simulink model "web_log"  (Simulink 7.3)
settings: Solver=ode3  SolverMode=SingleTasking  StartTime=0.0  StopTime=10.0  RelTol=1e-3
PreLoadFcn:
  | waijung.modelPreload; % Required for working with Waijung Blockset. Do not remove.
undefined symbols (not defined in the file): A0, A1, A2, A3, A7, B0, B1, B10, B11, B12, B13, Blocking, C1, C2, C3, C4, C5, HSEOSC, Link, LQFP176, Non, ST, STM32F417IG
libraries: simulink x45, amg_sqlite_dataserver x3, waijung_webserver x3, stm32f4_io_lib x1, stm32f4_device_config_lib x1
(part 1 of 3)
CloseFcn:
  | waijung.modelClose; % Required for working with Waijung Blockset. Do not remove.
settings Model: Creator=Krisada  LastModifiedBy=Krisada
settings OptimizationCC: OptimizeModelRefInitCode=on  LifeSpan=1
settings HardwareCC: ProdEndianess=LittleEndian  ProdHWDeviceType=ARM Compatible->Cortex - M4  TargetEndianess=LittleEndian  TargetHWDeviceType=ARM Compatible->Cortex - M4
settings RTWCC: SystemTargetFile=stm32f4.tlc  GenerateMakefile=off  TemplateMakefile=ert_default_tmf  Description=STM32F4 Target  ProcessScript=stm32f4_make_rtw_hook
settings CodeAppCC: IgnoreCustomStorageClasses=off
settings STFCustomTargetCC: ModelReferenceCompliant=off  CombineOutputUpdateFcns=on  ERTCustomFileBanners=on  SupportContinuousTime=off  SupportNonInlinedSFcns=off  SystemTargetFile=stm32f4.tlc
settings ERTTargetCC: MultiwordLength=2048  ModelReferenceCompliant=off  ParMdlRefBuildCompliant=off  CompOptLevelCompliant=off  ERTFirstTimeCompliant=off  ModelStepFunctionPrototypeControlCompliant=off  CPPClassGenCompliant=off  InlinedParameterPlacement=NonHierarchical  ERTSrcFileBannerTemplate=stm32f4_code_template.cgt  ERTHdrFileBannerTemplate=stm32f4_code_template.cgt  ERTDataSrcFileTemplate=stm32f4_code_template.cgt  ERTDataHdrFileTemplate=stm32f4_code_template.cgt  ERTCustomFileTemplate=stm32f4_file_process.tlc

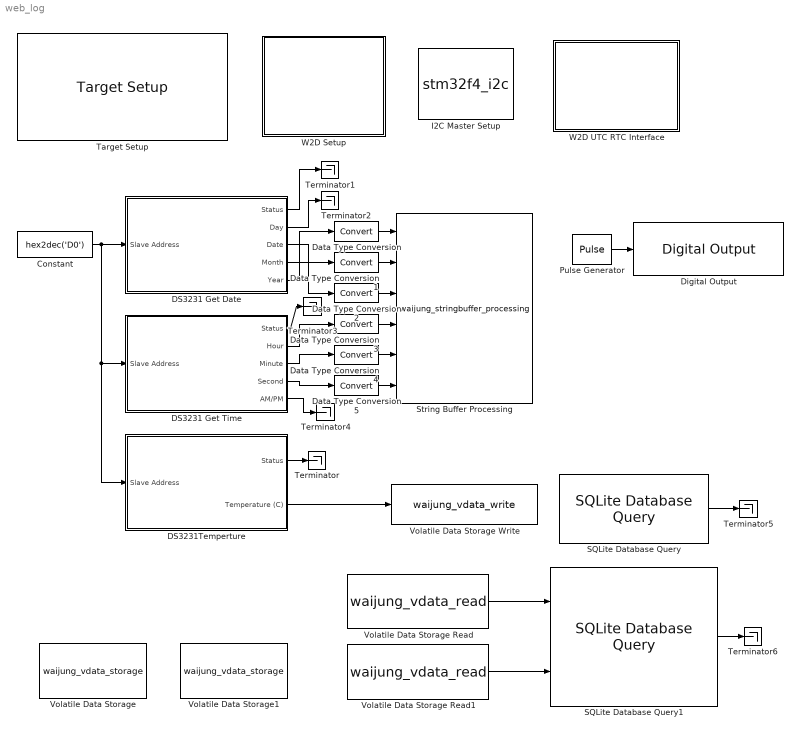
== system web_log ==
  Constant : Constant  Value=hex2dec('D0')  OutDataTypeMode=uint8  OutDataType=fixdt(1, 16)  OutScaling=2^0  OutDataTypeStr=uint8
  DS3231 Get Date : Subsystem  mask{blockfunction=date, module=1}
      mask prompts: blockfunction "Function"; module "I2C module"
      mask init:
      | amg_high_precision_rtc_callback('init');
      mask Help: web(fullfile(waijungdocroot,'DS3231_Get_Date.htm'), '-browser')
      mask StyleString: popup(temp|time|date),popup(1|2|3)
      mask CallbackString: |amg_high_precision_rtc_callback('module');
      mask Display: text(0.5, 0.5, 'Port: I2C1','ver','middle','hor','center');port_label('input', 1,'SlvAddr');port_label('output', 1,'Status');port_label('output', 2,'Day(1-7)');port_label('output', 3,'Date(1-31)');port_label('output', 4,'Month(1-12)');port_label('output', 5,'Year(0-99)');
  DS3231 Get Time : Subsystem  mask{blockfunction=time, module=1}
      mask prompts: blockfunction "Function"; module "I2C module"
      mask init:
      | amg_high_precision_rtc_callback('init');
      mask Help: web(fullfile(waijungdocroot,'DS3231_Get_Time.htm'), '-browser')
      mask StyleString: popup(temp|time|date),popup(1|2|3)
      mask CallbackString: |amg_high_precision_rtc_callback('module');
      mask Display: text(0.5, 0.5, 'Port: I2C1','ver','middle','hor','center');port_label('input', 1,'SlvAddr');port_label('output', 1,'Status');port_label('output', 2,'Hour(0-11/23)');port_label('output', 3,'Minute(0-59)');port_label('output', 4,'Second(0-59)');port_label('output', 5,'AM(0)/PM(1)');
  DS3231Temperture : Subsystem  mask{blockfunction=temp, module=1}
      mask prompts: blockfunction "Function"; module "I2C module"
      mask help:
      | The block implement temperature reading from DS3231 (Extremely Accurate RTC).
      | Its override the CONV bit, to force the temperature update, so the recommend sample time for this block is more than 0.5 seconds.
      | To get reading value from DS3231 device, this block generate 3 transaction of I2C as below:
      | 1. Read 2 bytes data from register 0x11 and 0x12 (Sequential read).
      | 2. Read 1 byte data from register 0x0F (Status) for poll BSY bit.
      | 3. Write 1 byte data to register 0x0E to force temperature conversion, CONV bit.
      mask init:
      | amg_high_precision_rtc_callback('init');
      mask Help: web(fullfile(waijungdocroot,'DS3231Temperture.htm'), '-browser')
      mask StyleString: popup(temp|time|date),popup(1|2|3)
      mask CallbackString: |amg_high_precision_rtc_callback('module');
      mask Display: text(0.5, 0.5, 'Port: I2C1','ver','middle','hor','center');port_label('input', 1,'SlvAddr');port_label('output', 1,'Status');port_label('output', 2,'Temp (C)');
  Data Type Conversion{,1..5} (6 alike) : DataTypeConversion  OutDataType=fixdt(1, 16)  OutScaling=2^0
  Digital Output : stm32f4_io_lib/Digital Output  use_bitband=on  port=D  speed=100  porttype=Push Pull  porttypestr=PP  use_pin0=off  use_pin1=off  use_pin2=off  use_pin3=off  use_pin4=off  use_pin5=off  use_pin6=off  use_pin7=off  use_pin8=off  use_pin9=off  use_pin10=off  use_pin11=off  use_pin12=on  use_pin13=off  use_pin14=off  use_pin15=off  pinstr=GPIO_Pin_12  usedpinarray="[0  0  0  0  0  0  0  0  0  0  0  0  1  0  0  0]"  bitbandingstr="#define DigitalOutput_D12 Peripheral_BB(GPIOD->ODR, 12)  /* Output pin */"  sampletime=-1  sampletimestr=0.25  blockid=DigitalOutput  enablecustomportlabel=off  globalinit=off  cinputportlabel=In1, In2  coutputportlabel=0
  I2C Master Setup : S-Function  FunctionName=stm32f4_i2c  Parameters=configuration,module,transfer,clkspeed,timeout,sdapin,sclpin,writecount,readcount,inputtypearray,outputtypearray,confstr,sampletime,sampletimestr,blockid  EnableBusSupport=off  mask(stm32f4_i2c){configuration=Setup, module=1, lastmodule=1, transfer=Blocking, dutycycle=TLow/THigh = 2, clkspeed=400, timeout=25, writecount=0, readcount=0, sdapin=B7, sclpin=B6, waitwritetime=0, inputtypearray=[0], outputtypearray=[0], confstr=["B","7","B","6","1","1","6","0","I2C_DutyCycle_2","0","off"], sampletime=-1, sampletimestr=0.001, blockid=I2CMasterSetup}
      mask prompts: module "I2C Module"; lastmodule "Last module"; transfer "Transfer mode"; dutycycle "Duty cycle in fast mode"; clkspeed "Clock speed (kHz)"; timeout "Timeout (ms)"; writecount "Bytes write count"; readcount "Bytes read count"; sdapin "SDA pin"; sclpin "SCL pin"; waitwritetime "Wait write time (ms), default is 0"; inputtypearray "Input type array"; outputtypearray "Output type array"; confstr "Configuration string"; sampletime "Sample time (sec)"; sampletimestr "Compiled sample time (sec) in string"
      mask init:
      | stm32f4_i2c_callback('init');
      mask Help: web(fullfile(waijungdocroot,'stm32f4_i2c_setup.htm'), '-browser')
      mask StyleString: popup(Setup|Transaction),popup(1|2|3),edit,popup(Blocking|Non-blocking),popup(TLow/THigh = 16/9|TLow/THigh = 2),edit,edit,edit,edit,popup(Not used|B7|B9),popup(Not used|B6|B8),edit,edit,edit,edit,edit,edit,edit
      mask CallbackString: stm32f4_i2c_callback('configuration');|stm32f4_i2c_callback('module');|||stm32f4_i2c_callback('dutycycle');|||stm32f4_i2c_callback('writecount');|stm32f4_i2c_callback('readcount');|stm32f4_i2c_callback('sdapin');|stm32f4_i2c_callback('sclpin');||||stm32f4_i2c_callback('confstr');|stm32f4_i2c_callback('sampletime');|stm32f4_i2c_callback('sampletimestr');|stm32f4_i2c_callback('blockid');
      mask Display: text(0.5, 0.5, 'Module: I2C1\nClock: 400kHz\nSDA/SCL Pin: B7/B6','ver','middle','hor','center');
  Pulse Generator : DiscretePulseGenerator  PulseType=Time based  Amplitude=1  Period=0.5  PulseWidth=50  PhaseDelay=0  SampleTime=1
  SQLite Database Query : amg_sqlite_dataserver/SQLite Database Query  Priority=1  transfer=Non-Blocking  statement=CREATE  filenameoption=Specific  filename='database.db'  tablenameoption=Specific  tablename='logging'  columns='time text,temp real'  condition='where rowid==1'  preview=CREATE TABLE IF NOT EXISTS %s(time text,temp real);  enablestatus=on  columncount=2  columnnamesarray="[\"time\",\"temp\"]"  columntypesarray="[\"string\",\"single\"]"  inputtypearray=[]  outputtypearray=[7]  sampletime=inf  sampletimestr=0.001  blockid=SQLiteDatabaseQuery
  SQLite Database Query1 : amg_sqlite_dataserver/SQLite Database Query  Priority=5  transfer=Non-Blocking  statement=INSERT  filenameoption=Specific  filename='database.db'  tablenameoption=Specific  tablename='logging'  columns='time text,temp real'  condition='where rowid==1'  preview=INSERT INTO %s (time,temp)VALUES('%s',%f);  enablestatus=on  columncount=2  columnnamesarray="[\"time\",\"temp\"]"  columntypesarray="[\"string\",\"single\"]"  inputtypearray=[7 1]  outputtypearray=[7]  sampletime=30  sampletimestr=30  blockid=SQLiteDatabaseQuery1
  String Buffer Processing : S-Function  Priority=1  FunctionName=waijung_stringbuffer_processing  Parameters=configuration,varname,sformat,porttypes,portcount,inputtypearray,outputtypearray,sampletime,sampletimestr,blockid  EnableBusSupport=off  mask(waijung_stringbuffer_processing){configuration=sprintf, storagename=timestring, sformat='%02d%02d%02d%02d%02d%02d', enableoutput=off, varname=VolatileDataStorage_timestring, inputtypearray=[6 -1 -1 -1 -1 -1 -1], outputtypearray=[0], porttypes=["int32_t","int32_t","int32_t","int32_t","int32_t","int32_t"], portcount=6, sampletime=1, sampletimestr=1, blockid=StringBufferProcessing}
      mask prompts: configuration "Function"; storagename "String buffer"; sformat "Printf format"; enableoutput "Enable output status"; varname "Variable name"; inputtypearray "Input type array"; outputtypearray "Output type array"; porttypes "Port type list"; portcount "Port type count"; sampletime "Sample time (sec)"; sampletimestr "Compiled sample time (sec) in string"
      mask help:
      | This block implements string processing, sprintf/ sscanf command.
      | Supported format:
      | %u, %i, %o, %x: uint32
      | %d: int32
      | %e, %g, %f: single
      | %c: int8
      |
      | Status:
      |  0: Failed.
      |  Non-zero: Success.
      mask init:
      | waijung_stringbuffer_processing_callback('init');
      mask Help: web(fullfile(waijungdocroot,'String_Buffer_Processing.htm'))
      mask StyleString: popup(sprintf|sscanf),popup(timestring|date|time|mcutime|browsertime|<output>),edit,checkbox,edit,edit,edit,edit,edit,edit,edit,edit
      mask CallbackString: waijung_stringbuffer_processing_callback('configuration');||waijung_stringbuffer_processing_callback('sformat');|waijung_stringbuffer_processing_callback('enableoutput');||||||waijung_stringbuffer_processing_callback('sampletime');|waijung_stringbuffer_processing_callback('sampletimestr');|waijung_stringbuffer_processing_callback('blockid');
      mask Display: text(0.5, 0.5, '[ sprintf ]\nBuffer: timestring\nTs (sec): 1','ver','middle','hor','center');port_label('input', 1,'%d');port_label('input', 2,'%d');port_label('input', 3,'%d');port_label('input', 4,'%d');port_label('input', 5,'%d');port_label('input', 6,'%d');
  Target Setup : stm32f4_device_config_lib/Target Setup  Priority=100  compiler=GNU ARM  previous_compiler=GNU ARM  mcu=STM32F417IG (LQFP176)  mcustr=STM32F417IG  clockconfig=HSEOSC-8MHz  system_stm32f4xx_c_path=F:\trunk\targets\stm32f4_target\stm32f4\utils\system_stm32f4xx_default\STM32F40_41xxx\hseosc8mhz  showmemoryconfiguration=on  stacksize=0x2000  heapsize=0x4000  enableautocompiledownload=on  fullchiperase=off  programmerinterface=ST-Link  editctrlstr=on  compilercontrolstr=$(patsubst %, -I%, .) -mcpu=cortex-m4 -mthumb -mthumb-interwork -mfloat-abi=hard -mfpu=fpv4-sp-d16 -ffast-math -Wall -Wextra -Ofast  assemblercontrolstr=$(patsubst %, -I%, .) -mcpu=cortex-m4 -mthumb -mthumb-interwork -mfloat-abi=hard -mfpu=fpv4-sp-d16 -ffast-math -Wall -Wextra -Ofast -Wa,-amhls=$(<:.s=.lst) -D__STACK_SIZE=$(STACK_SIZE) -D__HEAP_SIZE=$(HEAP_SIZE)  linkercontrolstr=-T$(LD_SCRIPT) -g -Wl,-Map=$(MAP),--cref,--no-warn-mismatch -mcpu=cortex-m4 -mthumb -mthumb-interwork -mfloat-abi=hard -mfpu=fpv4-sp-d16 -specs=nosys.specs  runafterdownload=on  execprofile=None  profileruart=3  profilerbaud=500000  profilertxpin=D8  profilerinitstr=0.001,168000000,168000,500000,0  manualsetsampletime=off  sampletime=0.001  blockid=TargetSetup  systickreloadvalue=168000  hseval=8000000  lastprofileruart=3  hclk=168000000  flashorigin=0x8000000  flashlength=1024k  ramorigin=0x20000000  ramlength=128k  useextram=off
  Terminator{,1..6} (7 alike) : Terminator
  Volatile Data Storage : S-Function  FunctionName=waijung_vdata_storage  Parameters=storagetype,storagename,initval,varname,buffersize,initvalstring,sampletime,sampletimestr,blockid,storagetypestr  EnableBusSupport=off  mask(waijung_vdata_storage){storagetype=string, storagename=timestring, initval=0, varname=VolatileDataStorage_timestring, buffersize=64, initvalstring='Initial string', webintegration=ReadOnly with KeyValuePair, weboutputformat='%s', webcgicallback=(void*)0, laststoragetype=string, sampletime=-1, sampletimestr=0.001, blockid=VolatileDataStorage, storagetypestr=char}
      mask prompts: storagetype "Storage Type"; storagename "Storage Name (must be a valid variable name)"; initval "Initial value (Apply at Power on Reset only)"; varname "Variable name"; buffersize "Size (bytes)"; initvalstring "Initial value (Apply at Power on Reset only)"; webintegration "Web CGI varget/varset integration"; weboutputformat "Web CGI varget output format"; webcgicallback "Web CGI varset callback"; laststoragetype "Last selected Storage Type"; sampletime "Sample time (sec)"; sampletimestr "Compiled sample time (sec) in string"; storagetypestr "Type string"
      mask help:
      | This block implements a volatile Data Storage.
      |
      | Web CGI varset/varget integratiopn:
      | Enable - In webserver application, allow remote access via http.
      | Disable - Variable is use in local only.
      mask init:
      | waijung_vdata_storage_callback('init');
      mask Help: web(fullfile(waijungdocroot,'Volatile_Data_Storage.htm'))
      mask StyleString: popup(double|single|uint32|int32|uint16|int16|uint8|int8|string),edit,edit,edit,edit,edit,popup(Disable|ReadOnly|Write/ Read|ReadOnly with KeyValuePair|Write/ Read with KeyValuePair),edit,edit,popup(double|single|uint32|int32|uint16|int16|uint8|int8|string),edit,edit,edit,edit
      mask CallbackString: waijung_vdata_storage_callback('storagetype');|waijung_vdata_storage_callback('storagename');|waijung_vdata_storage_callback('initval');|waijung_vdata_storage_callback('varname');||waijung_vdata_storage_callback('initvalstring');|waijung_vdata_storage_callback('webintegration');|waijung_vdata_storage_callback('weboutputformat');|||waijung_vdata_storage_callback('sampletime');|waijung_vdata_storage_callback('sampletimestr');|waijung_vdata_storage_callback('blockid');|
      mask Display: text(0.5, 0.5, 'Name: timestring\nType: string','ver','middle','hor','center')
  Volatile Data Storage Read : S-Function  FunctionName=waijung_vdata_read  Parameters=storagename,varname,sampletime,sampletimestr,blockid,storagetype,storagetypestr  EnableBusSupport=off  mask(waijung_vdata_read){storagename=timestring, varname=VolatileDataStorage_timestring, sampletime=inf, sampletimestr=30, blockid=VolatileDataStorageRead, storagetype=string, storagetypestr=uint32_t}
      mask prompts: storagename "Storage Name"; varname "Variable name"; sampletime "Sample time (sec)"; sampletimestr "Compiled sample time (sec) in string"; storagetype "Data type"; storagetypestr "Data type string"
      mask help: This block implements read data from a buffer.
      mask init:
      | waijung_vdata_read_callback('init');
      mask Help: web(fullfile(waijungdocroot,'Volatile_Data_Storage_Read.htm'))
      mask StyleString: popup(timestring|temperature|date|time|mcutime|browsertime|minth|hourth|secth),edit,edit,edit,edit,edit,edit
      mask CallbackString: waijung_vdata_read_callback('storagename');|waijung_vdata_read_callback('varname');|waijung_vdata_read_callback('sampletime');|waijung_vdata_read_callback('sampletimestr');|waijung_vdata_read_callback('blockid');|waijung_vdata_read_callback('storagetype');|
      mask Display: text(0.05, 0.5, 'Buffer: timestring','ver','middle','hor','left');port_label('output',1,'D1(string)')
  Volatile Data Storage Read1 : S-Function  FunctionName=waijung_vdata_read  Parameters=storagename,varname,sampletime,sampletimestr,blockid,storagetype,storagetypestr  EnableBusSupport=off  mask(waijung_vdata_read){storagename=temperature, varname=VolatileDataStorage1_temperature, sampletime=inf, sampletimestr=30, blockid=VolatileDataStorageRead1, storagetype=single, storagetypestr=float}
      mask prompts: storagename "Storage Name"; varname "Variable name"; sampletime "Sample time (sec)"; sampletimestr "Compiled sample time (sec) in string"; storagetype "Data type"; storagetypestr "Data type string"
      mask help: This block implements read data from a buffer.
      mask init:
      | waijung_vdata_read_callback('init');
      mask Help: web(fullfile(waijungdocroot,'Volatile_Data_Storage_Read.htm'))
      mask StyleString: popup(timestring|temperature|date|time|mcutime|browsertime|minth|hourth|secth),edit,edit,edit,edit,edit,edit
      mask CallbackString: waijung_vdata_read_callback('storagename');|waijung_vdata_read_callback('varname');|waijung_vdata_read_callback('sampletime');|waijung_vdata_read_callback('sampletimestr');|waijung_vdata_read_callback('blockid');|waijung_vdata_read_callback('storagetype');|
      mask Display: text(0.05, 0.5, 'Buffer: temperature','ver','middle','hor','left');port_label('output',1,'D1(single)')
  Volatile Data Storage Write : S-Function  FunctionName=waijung_vdata_write  Parameters=storagename,varname,sampletime,sampletimestr,blockid,storagetype,storagetypestr  EnableBusSupport=off  mask(waijung_vdata_write){storagename=temperature, varname=VolatileDataStorage1_temperature, sampletime=-1, sampletimestr=1, blockid=VolatileDataStorageWrite, storagetype=single, storagetypestr=float}
      mask prompts: storagename "Storage Name"; varname "Variable name"; sampletime "Sample time (sec)"; sampletimestr "Compiled sample time (sec) in string"; storagetype "Data type"; storagetypestr "Data type string"
      mask help: This block implements write data to a buffer.
      mask init:
      | waijung_vdata_write_callback('init');
      mask Help: web(fullfile(waijungdocroot,'Volatile_Data_Storage_Write.htm'))
      mask StyleString: popup(timestring|temperature|date|time|mcutime|browsertime|minth|hourth|secth),edit,edit,edit,edit,edit,edit
      mask CallbackString: waijung_vdata_write_callback('storagename');|waijung_vdata_write_callback('varname');|waijung_vdata_write_callback('sampletime');|waijung_vdata_write_callback('sampletimestr');|waijung_vdata_write_callback('blockid');|waijung_vdata_write_callback('storagetype');|
      mask Display: text(0.95, 0.5, 'Buffer: temperature','ver','middle','hor','right');port_label('input',1,'D1(single)')
  Volatile Data Storage1 : S-Function  FunctionName=waijung_vdata_storage  Parameters=storagetype,storagename,initval,varname,buffersize,initvalstring,sampletime,sampletimestr,blockid,storagetypestr  EnableBusSupport=off  mask(waijung_vdata_storage){storagetype=single, storagename=temperature, initval=0, varname=VolatileDataStorage1_temperature, buffersize=64, initvalstring='Initial string', webintegration=ReadOnly with KeyValuePair, weboutputformat='%f', webcgicallback=(void*)0, laststoragetype=single, sampletime=-1, sampletimestr=0.001, blockid=VolatileDataStorage1, storagetypestr=float}
      mask prompts: storagetype "Storage Type"; storagename "Storage Name (must be a valid variable name)"; initval "Initial value (Apply at Power on Reset only)"; varname "Variable name"; buffersize "Size (bytes)"; initvalstring "Initial value (Apply at Power on Reset only)"; webintegration "Web CGI varget/varset integration"; weboutputformat "Web CGI varget output format"; webcgicallback "Web CGI varset callback"; laststoragetype "Last selected Storage Type"; sampletime "Sample time (sec)"; sampletimestr "Compiled sample time (sec) in string"; storagetypestr "Type string"
      mask help:
      | This block implements a volatile Data Storage.
      |
      | Web CGI varset/varget integratiopn:
      | Enable - In webserver application, allow remote access via http.
      | Disable - Variable is use in local only.
      mask init:
      | waijung_vdata_storage_callback('init');
      mask Help: web(fullfile(waijungdocroot,'Volatile_Data_Storage.htm'))
      mask StyleString: popup(double|single|uint32|int32|uint16|int16|uint8|int8|string),edit,edit,edit,edit,edit,popup(Disable|ReadOnly|Write/ Read|ReadOnly with KeyValuePair|Write/ Read with KeyValuePair),edit,edit,popup(double|single|uint32|int32|uint16|int16|uint8|int8|string),edit,edit,edit,edit
      mask CallbackString: waijung_vdata_storage_callback('storagetype');|waijung_vdata_storage_callback('storagename');|waijung_vdata_storage_callback('initval');|waijung_vdata_storage_callback('varname');||waijung_vdata_storage_callback('initvalstring');|waijung_vdata_storage_callback('webintegration');|waijung_vdata_storage_callback('weboutputformat');|||waijung_vdata_storage_callback('sampletime');|waijung_vdata_storage_callback('sampletimestr');|waijung_vdata_storage_callback('blockid');|
      mask Display: text(0.5, 0.5, 'Name: temperature\nType: single','ver','middle','hor','center')
  W2D Setup : Subsystem
  W2D UTC RTC Interface : Subsystem  Priority=1
  wires:
  Pulse Generator/1 -> Digital Output/1
  Constant/1 -> DS3231 Get Date/1(Slave Address), DS3231 Get Time/1(Slave Address), DS3231Temperture/1(Slave Address)
  DS3231Temperture/1(Status) -> Terminator/1
  DS3231Temperture/2(Temperature (C)) -> Volatile Data Storage Write/1
  Data Type Conversion/1 -> String Buffer Processing/1
  Data Type Conversion1/1 -> String Buffer Processing/2
  Data Type Conversion2/1 -> String Buffer Processing/3
  Data Type Conversion3/1 -> String Buffer Processing/4
  Data Type Conversion4/1 -> String Buffer Processing/5
  Data Type Conversion5/1 -> String Buffer Processing/6
  DS3231 Get Date/5(Year) -> Data Type Conversion/1
  DS3231 Get Date/4(Month) -> Data Type Conversion1/1
  DS3231 Get Date/3(Date) -> Data Type Conversion2/1
  DS3231 Get Time/2(Hour) -> Data Type Conversion3/1
  DS3231 Get Time/3(Minute) -> Data Type Conversion4/1
  DS3231 Get Time/4(Second) -> Data Type Conversion5/1
  DS3231 Get Date/1(Status) -> Terminator1/1
  DS3231 Get Date/2(Day) -> Terminator2/1
  DS3231 Get Time/1(Status) -> Terminator3/1
  DS3231 Get Time/5(AM/PM) -> Terminator4/1
  SQLite Database Query/1 -> Terminator5/1
  SQLite Database Query1/1 -> Terminator6/1
  Volatile Data Storage Read/1 -> SQLite Database Query1/1
  Volatile Data Storage Read1/1 -> SQLite Database Query1/2

== system web_log/DS3231 Get Date ==
  Slave Address : Inport  OutDataType=fixdt(1, 16)  OutScaling=2^0
  Compare To Zero : simulink/Logic and Bit Operations/Compare To Zero  SystemSampleTime=-1  relop===  LogicOutDataTypeMode=uint8  ZeroCross=off
  Convert : Subsystem  TreatAsAtomicUnit=on
  I2C Master Read/Write : S-Function  FunctionName=stm32f4_i2c  Parameters=configuration,module,transfer,clkspeed,timeout,sdapin,sclpin,writecount,readcount,inputtypearray,outputtypearray,confstr,sampletime,sampletimestr,blockid  EnableBusSupport=off  mask(stm32f4_i2c){configuration=Transaction, module=1, lastmodule=3, transfer=Blocking, dutycycle=TLow/THigh = 2, clkspeed=400, timeout=25, writecount=1, readcount=4, sdapin=C9, sclpin=A8, waitwritetime=0, inputtypearray=[2 3 3], outputtypearray=[5 3 3 3 3 3], confstr=["C","9","A","8","1","1","6","0","I2C_DutyCycle_2","0","off"], sampletime=-1, sampletimestr=1, blockid=DS3231GetDateI2CMasterReadWrite}
      mask prompts: module "I2C Module"; lastmodule "Last module"; transfer "Transfer mode"; dutycycle "Duty cycle in fast mode"; clkspeed "Clock speed (kHz)"; timeout "Timeout (ms)"; writecount "Bytes write count"; readcount "Bytes read count"; sdapin "SDA pin"; sclpin "SCL pin"; waitwritetime "Wait write time (ms), default is 0"; inputtypearray "Input type array"; outputtypearray "Output type array"; confstr "Configuration string"; sampletime "Sample time (sec)"; sampletimestr "Compiled sample time (sec) in string"
      mask init:
      | stm32f4_i2c_callback('init');
      mask Help: web(fullfile(waijungdocroot,'stm32f4_i2c_readwrite.htm'), '-browser')
      mask StyleString: popup(Setup|Transaction),popup(1|2|3),edit,popup(Blocking|Non-blocking),popup(TLow/THigh = 16/9|TLow/THigh = 2),edit,edit,edit,edit,popup(-|C9),popup(-|A8),edit,edit,edit,edit,edit,edit,edit
      mask CallbackString: stm32f4_i2c_callback('configuration');|stm32f4_i2c_callback('module');|||stm32f4_i2c_callback('dutycycle');|||stm32f4_i2c_callback('writecount');|stm32f4_i2c_callback('readcount');|stm32f4_i2c_callback('sdapin');|stm32f4_i2c_callback('sclpin');||||stm32f4_i2c_callback('confstr');|stm32f4_i2c_callback('sampletime');|stm32f4_i2c_callback('sampletimestr');|stm32f4_i2c_callback('blockid');
      mask Display: text(0.5, 0.5, 'Module: I2C1\nTransfer: Blocking\nWrite: 1 bytes\nRead: 4 bytes\nTs (sec): 1','ver','middle','hor','center');port_label('input', 1,'SlvAddr');port_label('input', 2,'Wr0 (uint8)');port_label('output', 1,'Status');port_label('output', 2,'Rd0 (uint8)');port_label('output', 3,'Rd1 (uint8)');port_label('output', 4,'Rd2 (uint8)');port_label('output', 5,'Rd3 (uint8)');
  REG_DATE : Constant  Value=hex2dec('03')  OutDataTypeMode=uint8  OutDataType=fixdt(1, 16)  OutScaling=2^0  OutDataTypeStr=uint8
  Status : Outport
  Day : Outport  Port=2
  Date : Outport  Port=3
  Month : Outport  Port=4
  Year : Outport  Port=5
  wires:
  Convert/3(Month) -> Month/1
  Convert/4(Year) -> Year/1
  Convert/2(Date) -> Date/1
  Convert/1(Day) -> Day/1
  I2C Master Read/Write/5 -> Convert/4(In4)
  REG_DATE/1 -> I2C Master Read/Write/2
  Slave Address/1 -> I2C Master Read/Write/1
  I2C Master Read/Write/1 -> Compare To Zero/1
  Compare To Zero/1 -> Convert/Enable, Status/1
  I2C Master Read/Write/2 -> Convert/1(In1)
  I2C Master Read/Write/3 -> Convert/2(In2)
  I2C Master Read/Write/4 -> Convert/3(In3)

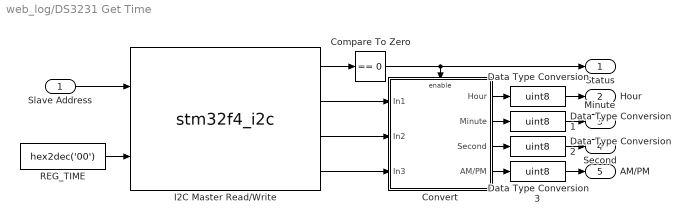
== system web_log/DS3231 Get Time ==
  Slave Address : Inport  OutDataType=fixdt(1, 16)  OutScaling=2^0
  Compare To Zero : simulink/Logic and Bit Operations/Compare To Zero  SystemSampleTime=-1  relop===  LogicOutDataTypeMode=uint8  ZeroCross=off
  Convert : Subsystem  TreatAsAtomicUnit=on
  Data Type Conversion{,1..3} (4 alike) : DataTypeConversion  OutDataTypeMode=uint8  OutDataType=fixdt(1, 16)  OutScaling=2^0  OutDataTypeStr=uint8
  I2C Master Read/Write : S-Function  FunctionName=stm32f4_i2c  Parameters=configuration,module,transfer,clkspeed,timeout,sdapin,sclpin,writecount,readcount,inputtypearray,outputtypearray,confstr,sampletime,sampletimestr,blockid  EnableBusSupport=off  mask(stm32f4_i2c){configuration=Transaction, module=1, lastmodule=3, transfer=Blocking, dutycycle=TLow/THigh = 2, clkspeed=400, timeout=25, writecount=1, readcount=3, sdapin=C9, sclpin=A8, waitwritetime=0, inputtypearray=[2 3 3], outputtypearray=[4 3 3 3 3], confstr=["C","9","A","8","1","1","6","0","I2C_DutyCycle_2","0","off"], sampletime=-1, sampletimestr=1, blockid=DS3231GetTimeI2CMasterReadWrite}
      mask prompts: module "I2C Module"; lastmodule "Last module"; transfer "Transfer mode"; dutycycle "Duty cycle in fast mode"; clkspeed "Clock speed (kHz)"; timeout "Timeout (ms)"; writecount "Bytes write count"; readcount "Bytes read count"; sdapin "SDA pin"; sclpin "SCL pin"; waitwritetime "Wait write time (ms), default is 0"; inputtypearray "Input type array"; outputtypearray "Output type array"; confstr "Configuration string"; sampletime "Sample time (sec)"; sampletimestr "Compiled sample time (sec) in string"
      mask init:
      | stm32f4_i2c_callback('init');
      mask Help: web(fullfile(waijungdocroot,'stm32f4_i2c_readwrite.htm'), '-browser')
      mask StyleString: popup(Setup|Transaction),popup(1|2|3),edit,popup(Blocking|Non-blocking),popup(TLow/THigh = 16/9|TLow/THigh = 2),edit,edit,edit,edit,popup(-|C9),popup(-|A8),edit,edit,edit,edit,edit,edit,edit
      mask CallbackString: stm32f4_i2c_callback('configuration');|stm32f4_i2c_callback('module');|||stm32f4_i2c_callback('dutycycle');|||stm32f4_i2c_callback('writecount');|stm32f4_i2c_callback('readcount');|stm32f4_i2c_callback('sdapin');|stm32f4_i2c_callback('sclpin');||||stm32f4_i2c_callback('confstr');|stm32f4_i2c_callback('sampletime');|stm32f4_i2c_callback('sampletimestr');|stm32f4_i2c_callback('blockid');
      mask Display: text(0.5, 0.5, 'Module: I2C1\nTransfer: Blocking\nWrite: 1 bytes\nRead: 3 bytes\nTs (sec): 1','ver','middle','hor','center');port_label('input', 1,'SlvAddr');port_label('input', 2,'Wr0 (uint8)');port_label('output', 1,'Status');port_label('output', 2,'Rd0 (uint8)');port_label('output', 3,'Rd1 (uint8)');port_label('output', 4,'Rd2 (uint8)');
  REG_TIME : Constant  Value=hex2dec('00')  OutDataTypeMode=uint8  OutDataType=fixdt(1, 16)  OutScaling=2^0  OutDataTypeStr=uint8
  Status : Outport
  Hour : Outport  Port=2
  Minute : Outport  Port=3
  Second : Outport  Port=4
  AM/PM : Outport  Port=5
  wires:
  Data Type Conversion3/1 -> AM/PM/1
  Data Type Conversion2/1 -> Second/1
  Data Type Conversion1/1 -> Minute/1
  Data Type Conversion/1 -> Hour/1
  Convert/4(AM/PM) -> Data Type Conversion3/1
  Convert/1(Hour) -> Data Type Conversion/1
  Convert/2(Minute) -> Data Type Conversion1/1
  Convert/3(Second) -> Data Type Conversion2/1
  I2C Master Read/Write/4 -> Convert/3(In3)
  I2C Master Read/Write/3 -> Convert/2(In2)
  I2C Master Read/Write/2 -> Convert/1(In1)
  Compare To Zero/1 -> Status/1, Convert/Enable
  I2C Master Read/Write/1 -> Compare To Zero/1
  Slave Address/1 -> I2C Master Read/Write/1
  REG_TIME/1 -> I2C Master Read/Write/2

== system web_log/DS3231Temperture ==
  Slave Address : Inport  OutDataType=fixdt(1, 16)  OutScaling=2^0
  Check Busy/ Write Conv : Subsystem
  Compare To Zero : simulink/Logic and Bit Operations/Compare To Zero  SystemSampleTime=-1  relop===  LogicOutDataTypeMode=uint8  ZeroCross=off
  Convert : Subsystem  TreatAsAtomicUnit=on
  I2C Master Read/Write : S-Function  FunctionName=stm32f4_i2c  Parameters=configuration,module,transfer,clkspeed,timeout,sdapin,sclpin,writecount,readcount,inputtypearray,outputtypearray,confstr,sampletime,sampletimestr,blockid  EnableBusSupport=off  mask(stm32f4_i2c){configuration=Transaction, module=1, lastmodule=3, transfer=Blocking, dutycycle=TLow/THigh = 2, clkspeed=400, timeout=25, writecount=1, readcount=2, sdapin=C9, sclpin=A8, waitwritetime=0, inputtypearray=[2 3 3], outputtypearray=[3 3 3 3], confstr=["C","9","A","8","1","1","6","0","I2C_DutyCycle_2","0","off"], sampletime=-1, sampletimestr=1, blockid=DS3231TempertureI2CMasterReadWrite}
      mask prompts: module "I2C Module"; lastmodule "Last module"; transfer "Transfer mode"; dutycycle "Duty cycle in fast mode"; clkspeed "Clock speed (kHz)"; timeout "Timeout (ms)"; writecount "Bytes write count"; readcount "Bytes read count"; sdapin "SDA pin"; sclpin "SCL pin"; waitwritetime "Wait write time (ms), default is 0"; inputtypearray "Input type array"; outputtypearray "Output type array"; confstr "Configuration string"; sampletime "Sample time (sec)"; sampletimestr "Compiled sample time (sec) in string"
      mask init:
      | stm32f4_i2c_callback('init');
      mask Help: web(fullfile(waijungdocroot,'stm32f4_i2c_readwrite.htm'), '-browser')
      mask StyleString: popup(Setup|Transaction),popup(1|2|3),edit,popup(Blocking|Non-blocking),popup(TLow/THigh = 16/9|TLow/THigh = 2),edit,edit,edit,edit,popup(-|C9),popup(-|A8),edit,edit,edit,edit,edit,edit,edit
      mask CallbackString: stm32f4_i2c_callback('configuration');|stm32f4_i2c_callback('module');|||stm32f4_i2c_callback('dutycycle');|||stm32f4_i2c_callback('writecount');|stm32f4_i2c_callback('readcount');|stm32f4_i2c_callback('sdapin');|stm32f4_i2c_callback('sclpin');||||stm32f4_i2c_callback('confstr');|stm32f4_i2c_callback('sampletime');|stm32f4_i2c_callback('sampletimestr');|stm32f4_i2c_callback('blockid');
      mask Display: text(0.5, 0.5, 'Module: I2C1\nTransfer: Blocking\nWrite: 1 bytes\nRead: 2 bytes\nTs (sec): 1','ver','middle','hor','center');port_label('input', 1,'SlvAddr');port_label('input', 2,'Wr0 (uint8)');port_label('output', 1,'Status');port_label('output', 2,'Rd0 (uint8)');port_label('output', 3,'Rd1 (uint8)');
  REG_TEMP : Constant  Value=hex2dec('11')  OutDataTypeMode=uint8  OutDataType=fixdt(1, 16)  OutScaling=2^0  OutDataTypeStr=uint8
  Status : Outport
  Temperature (C) : Outport  Port=2
  wires:
  Convert/1(Reading) -> Temperature (C)/1
  I2C Master Read/Write/3 -> Convert/2(In2)
  I2C Master Read/Write/2 -> Convert/1(In1)
  Compare To Zero/1 -> Check Busy/ Write Conv/Enable, Convert/Enable
  I2C Master Read/Write/1 -> Compare To Zero/1, Status/1
  REG_TEMP/1 -> I2C Master Read/Write/2
  Slave Address/1 -> Check Busy/ Write Conv/1(In1), I2C Master Read/Write/1

== system web_log/W2D Setup ==
  Ethernet Application Setup : waijung_webserver/Ethernet Application Setup  conf=Setup  ipaddress=192.168.1.30  netmask=255.255.255.0  gateway=192.168.1.1  macaddress=02-00-00-00-00-00  dhcp=off  timerscaler=10  portpinstr=0  sampletime=0.001  blockid=W2DSetupEthernetApplicationSetup  inputporttype=[]  inputportwidth=[]  inputportlabel={}  outputporttype=[]  outputportwidth=[]  outputportlabel={}  compat=0  optionstring="[\"Dummy\",\"192\",\"168\",\"1\",\"30\",\"255\",\"255\",\"255\",\"0\",\"192\",\"168\",\"1\",\"1\",\"02\",\"00\",\"00\",\"00\",\"00\",\"00\",\"off\",\"10\"]"
  Ethernet Link Setup : waijung_webserver/Ethernet Link Setup  conf=Setup  interfacepin=Profile #1  wj_interfacetype=MII  pin_mdio=A2  pin_mdc=C1  pin_pps=Not used  pin_crs=A0  pin_col=A3  pin_dv=A7  pin_rxclk=A1  pin_rxer=B10  pin_rxd0=C4  pin_rxd1=C5  pin_rxd2=B0  pin_rxd3=B1  pin_txclk=C3  pin_txen=B11  pin_txd0=B12  pin_txd1=B13  pin_txd2=C2  pin_txd3=E2  portpinstr=A0,A1,A2,A3,A7,B0,B1,E2,B10,B11,B12,B13,C1,C2,C3,C4,C5  sampletime=inf  blockid=W2DSetupEthernetLinkSetup  inputporttype=[]  inputportwidth=[]  inputportlabel={}  outputporttype=[]  outputportwidth=[]  outputportlabel={}  compat=0  optionstring="[\"xxx\",\"on\",\"on\",\"on\",\"off\",\"on\",\"off\",\"off\",\"off\",\"off\",\"on\",\"on\",\"on\",\"on\",\"on\",\"on\",\"on\",\"off\",\"on\",\"on\",\"on\",\"on\",\"on\",\"on\",\"on\",\"on\",\"on\",\"on\",\"A\",\"0\",\"A\",\"1\",\"A\",\"2\",\"A\",\"3\",\"A\",\"7\",\"B\",\"0\",\"B\",\"1\",\"N\",\"ot used\",\"E\",\"2\",\"B\",\"10\",\"B\",\"11\",\"B\",\"12\",\"B\",\"13\",\"C\",\"1\",\"C\",\"2\",\"C\",\"3\",\"C\",\"4\",\"C\",\"5\",\"MII\"]"
  Http Server Setup : waijung_webserver/Http Server Setup  conf=Setup  port=80  ssl=Disable  sqlite=Enable  iap=Disable  mempool=8  debugport=Disable  portpinstr=0  sampletime=inf  blockid=W2DSetupHttpServerSetup  inputporttype=[]  inputportwidth=[]  inputportlabel={}  outputporttype=[]  outputportwidth=[]  outputportlabel={}  compat=0  optionstring="[\"80\",\"0\",\"0\",\"Enable\",\"Disable\",\"8\",\"17.02a\",\"\",\"\",\"\",\"timestring\",\"string\",\"VolatileDataStorage_timestring\",\"64\",\"0\",\"1\",\"(void*)0\",\"%s\",\"\",\"\",\"temperature\",\"single\",\"VolatileDataStorage1_temperature\",\"1\",\"0\",\"1\",\"(void*)0\",\"%f\",\"\",\"\",\"date\",\"string\",\"W2DUTCRTCInterfaceVolatileDataStorage1_date\",\"64\",\"0\",\"1\",\"(void*)0\",\"%s\",\"\",\"\",\"time\",\"string\",\"W2DUTCRTCInterfaceVolatileDataStorage2_time\",\"64\",\"0\",\"1\",\"(void*)0\",\"%s\",\"\",\"\",\"mcutime\",\"string\",\"W2DUTCRTCInterfaceVolatileDataStorage3_mcutime\",\"64\",\"0\",\"1\",\"(void*)0\",\"%s\",\"\",\"\",\"browsertime\",\"string\",\"W2DUTCRTCInterfaceVolatileDataStorage4_browsertime\",\"64\",\"1\",\"1\",\"W2DUTCRTCInterfaceHttpserverCGIvarsetcallback_varset_ISR\",\"%s\",\"\",\"\",\"minth\",\"int32\",\"W2DUTCRTCInterfaceVolatileDataStorage5_minth\",\"1\",\"0\",\"1\",\"(void*)0\",\"%d\",\"\",\"\",\"hourth\",\"int32\",\"W2DUTCRTCInterfaceVolatileDataStorage6_hourth\",\"1\",\"0\",\"1\",\"(void*)0\",\"%d\",\"\",\"\",\"secth\",\"int32\",\"W2DUTCRTCInterfaceVolatileDataStorage7_secth\",\"1\",\"0\",\"1\",\"(void*)0\",\"%d\",\"\",\"\"]"
  SQLite Database Setup : amg_sqlite_dataserver/SQLite Database Setup  Priority=1  port=UART6  timeout=5  buffersize=8192  reset=Software  resetport=A  resetpin=0  inputtypearray=[0]  outputtypearray=[0]  sampletime=inf  sampletimestr=0.001  blockid=W2DSetupSQLiteDatabaseSetup
  UART Setup : S-Function  Priority=1  FunctionName=stm32f4_usart  Parameters=configuration,uartmodule,transfer,baudrate,inputtype,outputtype,confstr,binheaderarray,binterminatorarray,asciiheader,asciiterminator,bindatalength,packetmode,varname,sampletime,sampletimestr,blockid  EnableBusSupport=off  mask(stm32f4_usart){configuration=Setup, uartmodule=6, baudrate=1e6, databits=8, parity=No, stopbit=1, remaptxpin=C6, remaprxpin=C7, flowcontrol=None, remapctspin=Not used, remaprtspin=Not used, advanceoptions=on, rxbuffersize=2048, txbuffersize=1024, transfer=Blocking, packetmode=Ascii, binheader='7E 7E', binterminator='03 03', porttype_double=1, porttype_single=0, porttype_int8=1, porttype_uint8=0, porttype_int16=0, porttype_uint16=0, porttype_int32=0, porttype_uint32=0, asciiformat='%d,%f', rx_asciiterminator=CRLF (0x0D 0x0A - "\r\n"), tx_asciiterminator=CR (0x0D - "\r"), storagename=<empty>, varname=, inputtype=[0], outputtype=[0], binheaderarray=[0], binterminatorarray=[0], bindatalength=0, asciiheader='', asciiterminator=[0], sampletime=-1, sampletimestr=0.001, blockid=W2DSetupUARTSetup, confstr=[ "dummy", "1", "C", "6", "1", "C", "7", "0", "*", "*", "0", "*", "*", "2", "5", "6", "2", "5", "1", "1024", "2048", "2", "6", "1e6", "8", "No", "1", "None", "USART6"], lastmodule=6}
      mask prompts: uartmodule "UART Module"; baudrate "Baud rate (bps)"; databits "Data bits"; stopbit "Stop bit"; remaptxpin "Tx Pin"; remaprxpin "Rx Pin"; flowcontrol "Hardware flow control"; remapctspin "HW Flow control, CTS Pin"; remaprtspin "HW Flow control, RTS Pin"; advanceoptions "Advance options"; rxbuffersize "Rx buffer size (bytes)"; txbuffersize "Tx buffer size (bytes)"; packetmode "Packet mode"; binheader "Binary header (example: '7E 7E')"; binterminator "Binary terminator (example: '03 03')"; porttype_double "Number of data port, type DOUBLE"; porttype_single "Number of data port, type SINGLE"; porttype_int8 "Number of data port, type INT8"; porttype_uint8 "Number of data port, type UINT8"; porttype_int16 "Number of data port, type INT16"; porttype_uint16 "Number of data port, type UINT16"; porttype_int32 "Number of data port, type INT32"; porttype_uint32 "Number of data port, type UINT32"; asciiformat "Ascii format"; rx_asciiterminator "End of packet"; tx_asciiterminator "End of packet"; storagename "Buffer"; varname "Var name"; inputtype "Input data type"; outputtype "Output data type"; binheaderarray "Binary header"; binterminatorarray "Binary terminator"; bindatalength "Binary data length"; asciiheader "Ascii header (printf format)"; asciiterminator "Ascii terminator"; sampletime "Sample time (sec)"; sampletimestr "Compiled sample time (sec) in string"; confstr "Configuration string"; lastmodule "Last module selected"
      mask init:
      | stm32f4_usart_callback('init');
      mask Help: web(fullfile(waijungdocroot,'stm32f4_usart_setup.htm'), '-browser')
      mask StyleString: popup(Setup|Tx|Rx),popup(1|2|3|4|5|6),edit,popup(8),popup(No|Odd|Even),popup(0.5|1|1.5|2),popup(Not used|C6|G14),popup(Not used|C7|G9),popup(None|RTS|CTS|RTS/CTS),popup(Not used|G13|G15),popup(Not used|G8|G12),checkbox,popup(16|32|64|128|256|512|1024|2048),popup(16|32|64|128|256|512|1024|2048),popup(Blocking|Non-Blocking),popup(Ascii|Binary|String Buffer),edit,edit,edit,edit,edit,edit,edit,edit,edit,edit,edit,popup(CR (0x0D - "\r")|LF (0x0A - "\n")|CRLF (0x0D 0x0A - "\r\n")),popup(CR (0x0D - "\r")|LF (0x0A - "\n")|CRLF (0x0D 0x0A - "\r\n")|None),popup(<empty>),edit,edit,edit,edit,edit,edit,edit,edit,edit,edit,edit,edit,edit
      mask CallbackString: stm32f4_usart_callback('configuration');|stm32f4_usart_callback('uartmodule');|stm32f4_usart_callback('baudrate');||||||stm32f4_usart_callback('flowcontrol');|||stm32f4_usart_callback('advanceoptions');|||stm32f4_usart_callback('transfer');|stm32f4_usart_callback('packetmode');|stm32f4_usart_callback('binheader');|stm32f4_usart_callback('binterminator');|stm32f4_usart_callback('porttype');|stm32f4_usart_callback('porttype');|stm32f4_usart_callback('porttype');|stm32f4_usart_callback('porttype');|stm32f4_usart_callback('porttype');|stm32f4_usart_callback('porttype');|stm32f4_usart_callback('porttype');|stm32f4_usart_callback('porttype');|stm32f4_usart_callback('asciiformat');|stm32f4_usart_callback('rx_asciiterminator');|stm32f4_usart_callback('tx_asciiterminator');|stm32f4_usart_callback('storagename');|stm32f4_usart_callback('varname');||||||||stm32f4_usart_callback('sampletime');|stm32f4_usart_callback('sampletimestr');|stm32f4_usart_callback('blockid');||
      mask Display: text(0.5, 0.5, 'Module: USART6_Setup\nBaud (Bps): 1e6\nDMA Buffer: 1024/2048\nTx/Rx Pin: C6/C7','ver','middle','hor','center');
